simulink model "ad_pmsm_or"  (R2022b)
settings: Solver=FixedStepAuto  StartTime=0.0  StopTime=0.6  FixedStep=5e-7  MaxStep=1e-5  RelTol=1e-4
InitFcn:
  | Ts = 10e-6;
  | 
  | R = 0.958;
  | Ld = 5.25e-3;
  | Lq = 12e-3;
  | Pn = 4;
  | flux = 0.1827;
undefined symbols (not defined in the file): b0_d, DiscIntNeverNeededParam
libraries: simulink x12, slpidlib x7, spsPermanentMagnetSynchronousMachineLib x4, spsUniversalBridgeLib x4, spsDCVoltageSourceLib x4, powerlib_extras x2, sps_lib x1
(part 1 of 3)
settings Model: Creator=SUN  LastModifiedBy=崔波
settings SolverCC: ZeroCrossControl=DisableAll  AlgebraicLoopSolver=TrustRegion  AutoInsertRateTranBlk=on
settings DataIOCC: LimitDataPoints=on  SaveFormat=Array  SignalLoggingSaveFormat=ModelDataLogs  ReturnWorkspaceOutputs=off
settings OptimizationCC: ExpressionDepthLimit=2147483647  InitFltsAndDblsToZero=on  LifeSpan=inf
settings DebuggingCC: UnderspecifiedInitializationDetection=Classic  MergeDetectMultiDrivingBlocksExec=none  SolverPrmCheckMsg=warning  MultiTaskRateTransMsg=warning  FcnCallInpInsideContextMsg=warning  UnconnectedInputMsg=warning  UnconnectedOutputMsg=warning  UnconnectedLineMsg=warning  StateNameClashWarn=warning  SFUnexpectedBacktrackingDiag=warning  SFNoUnconditionalDefaultTransitionDiag=warning  SFExecutionAtInitializationDiag=none  SFMachineParentedDataDiag=warning  ArithmeticOperatorsInVariantConditions=warning
settings HardwareCC: ProdBitPerPointer=32  ProdBitPerSizeT=32  ProdBitPerPtrDiffT=32  ProdLargestAtomicFloat=None  ProdIntDivRoundTo=Undefined  ProdEndianess=Unspecified  ProdWordSize=32  ProdHWDeviceType=32-bit Generic
settings ModelReferenceCC: PropagateSignalLabelsOutOfModel=off
settings SFSimCC: SimUseLocalCustomCode=off  CustomCodeUndefinedFunction=UseInterfaceOnly
settings RTWCC: RTWUseLocalCustomCode=off
settings CodeAppCC: StateflowObjectComments=on
settings GRTTargetCC: TargetLangStandard=C89/C90 (ANSI)  CombineOutputUpdateFcns=off  GRTInterface=on
settings ConfigComp: CovMetricSettings=dw  CovSaveCumulativeToWorkspaceVar=on  CovSaveSingleToWorkspaceVar=on  CovExternalEMLEnable=off  CovSFcnEnable=off
settings SimscapeCC: SimscapeNormalizeSystem=off

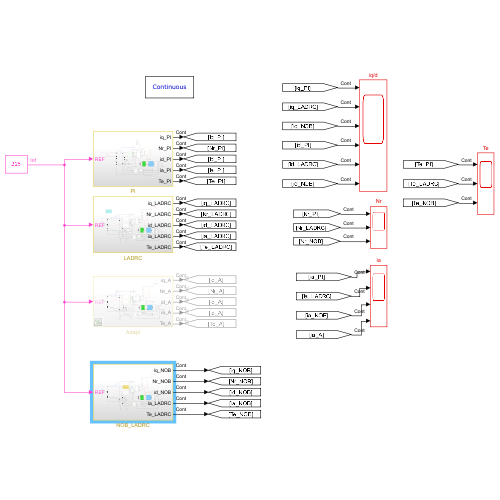
[thumbnail: Simulink's stored preview of the top-level diagram]
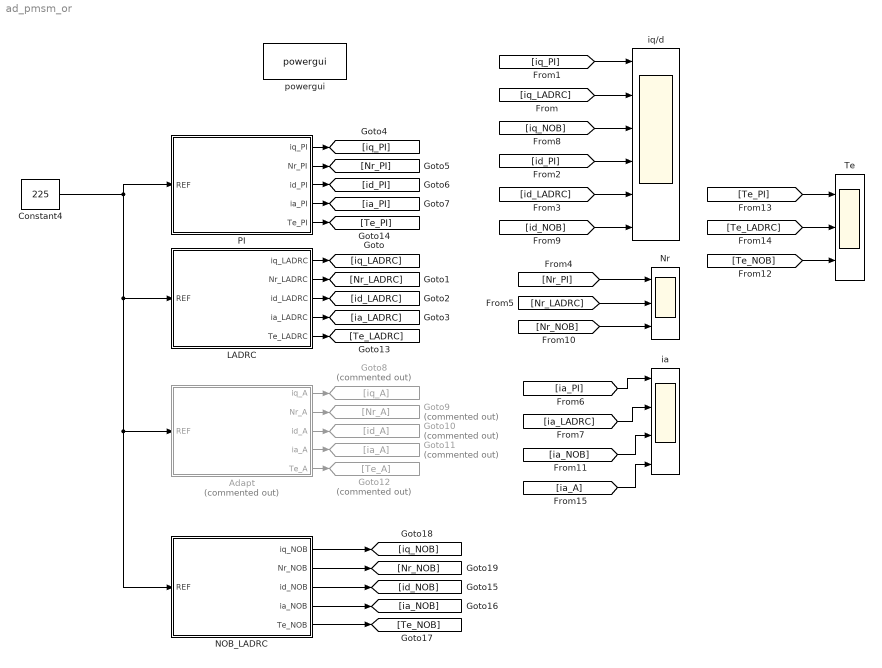
== system ad_pmsm_or ==
  Adapt : Subsystem  Commented=on
  Constant4 : Constant  Value=225
  Goto10 : Goto  Commented=on  GotoTag=id_A
  Goto11 : Goto  Commented=on  GotoTag=ia_A
  Goto12 : Goto  Commented=on  GotoTag=Te_A
  Goto8 : Goto  Commented=on  GotoTag=iq_A
  Goto9 : Goto  Commented=on  GotoTag=Nr_A
  LADRC : Subsystem
  NOB_LADRC : Subsystem
  Nr : Scope  NumInputPorts=3
  PI : Subsystem
  Te : Scope  NumInputPorts=3
  ia : Scope  NumInputPorts=4
  iq/d : Scope  NumInputPorts=6
  powergui : sps_lib/powergui  SimulationMode=Continuous  SampleTime=Ts  frequency=60  Iterations=50  frequencyindice=0  Pbase=100e6  ErrMax=1e-4  UnitsV=kV  UnitsW=MW  buscounter=0  FunctionMessages=off  echomessages=off  EnableUseOfTLC=off  CurrentSourceSwitches=on  DisableSnubberDevices=off  DisableRonSwitches=off  DisableVfSwitches=off  DisplayEquations=off  AutomaticDiscreteSolvers=off  SolverType=Tustin/Backward Euler (TBE)  Interpol=off  ExternalGateDelay=off  methode=off  Ts=0  x0status=blocks  SPID=off  SwTol=0  HookPort=off  NonlinearTolerance=1e-4  nMaxIteration=100  ContinueOnMaxIteration=off  RestoreLinks=warning  ResistiveCurrentMeasurement=off  Frange=[0:2:500]  Ylog=off  Xlog=on  ShowGrid=off  save=off  variable=ZData  structure=0  ZoomFFT=on  StartTime=0.0  cycles=1  DisplayStyle=1  fundamental=60  FreqAxis=off  MaxFrequency=1000  frequencyindicesteady=1  RmsSteady=1  display=off
  wires:
  LADRC/1(iq_LADRC) -> [iq_LADRC]
  LADRC/2(Nr_LADRC) -> [Nr_LADRC]
  LADRC/3(id_LADRC) -> [id_LADRC]
  LADRC/4(ia_LADRC) -> [ia_LADRC]
  [iq_PI] -> iq/d/1
  [id_PI] -> iq/d/4
  [id_LADRC] -> iq/d/5
  PI/2(Nr_PI) -> [Nr_PI]
  PI/4(ia_PI) -> [ia_PI]
  PI/3(id_PI) -> [id_PI]
  PI/1(iq_PI) -> [iq_PI]
  [Nr_PI] -> Nr/1
  [Nr_LADRC] -> Nr/2
  [ia_PI] -> ia/1
  [ia_LADRC] -> ia/2
  Adapt/2(Nr_A) -> Goto9/1
  Adapt/3(id_A) -> Goto10/1
  Constant4/1 -> NOB_LADRC/1(REF), Adapt/1(REF), LADRC/1(REF), PI/1(REF)
  Adapt/4(ia_A) -> Goto11/1
  Adapt/1(iq_A) -> Goto8/1
  [iq_NOB] -> iq/d/3
  [id_NOB] -> iq/d/6
  [Nr_NOB] -> Nr/3
  [ia_NOB] -> ia/3
  [Te_PI] -> Te/1
  [Te_LADRC] -> Te/2
  [Te_NOB] -> Te/3
  Adapt/5(Te_A) -> Goto12/1
  LADRC/5(Te_LADRC) -> [Te_LADRC]
  PI/5(Te_PI) -> [Te_PI]
  [iq_LADRC] -> iq/d/2
  NOB_LADRC/1(iq_NOB) -> [iq_NOB]
  NOB_LADRC/2(Nr_NOB) -> [Nr_NOB]
  NOB_LADRC/3(id_NOB) -> [id_NOB]
  NOB_LADRC/4(ia_NOB) -> [ia_NOB]
  NOB_LADRC/5(Te_NOB) -> [Te_NOB]
  [ia_A] -> ia/4

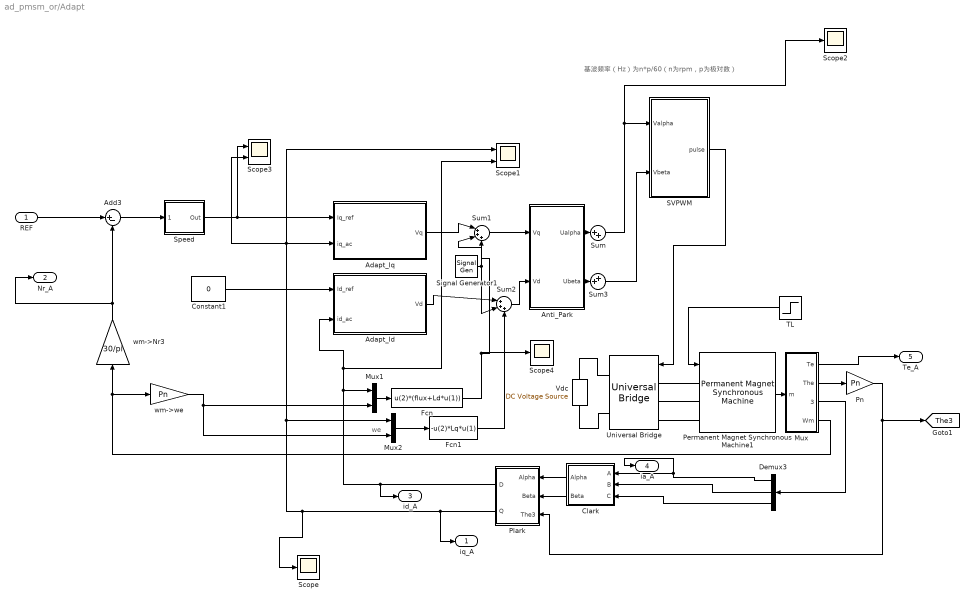
== system ad_pmsm_or/Adapt ==
  note: 基波频率（Hz）为n*p/60（n为rpm，p为极对数）
  note: we
  REF : Inport
  Adapt_Id : Subsystem  mask{Cd_l3=0.29, C_Krd=0.3, Ked=6.5, bd0=1/5.25e-3, wc_d=1100, wo_d=1100*3}
      mask DialogControl DescTextVar Prompt: 自适应谐振自抗扰控制器
      mask DialogControl ParameterGroupVar Prompt: 自抗扰控制器
      mask DialogControl Container3 Prompt: 自适应谐振控制器
      mask DialogControl Container4 Prompt: 频率自适应率
  Adapt_Iq : Subsystem  mask{bq0=1/12e-3, wc_q=1100, wo_q=1100*3, Cq_l3=0.29, C_Krq=0.3, Keq=0.3}
      mask DialogControl DescTextVar Prompt: 自适应谐振自抗扰控制器
      mask DialogControl ParameterGroupVar Prompt: 自抗扰控制器
      mask DialogControl Container3 Prompt: 自适应谐振控制器
      mask DialogControl Container4 Prompt: 频率自适应率
  Add3 : Sum  Inputs=|+-
  Anti_Park : Subsystem
  Clark : Subsystem
  Constant1 : Constant  Value=0
  Demux3 : Demux  Outputs=3
  Fcn : Fcn  Expr=u(2)*(flux+Ld*u(1))
  Fcn1 : Fcn  Expr=-u(2)*Lq*u(1)
  Mux : Subsystem
  Mux1 : Mux  Inputs=2
  Mux2 : Mux  Inputs=2
  Permanent Magnet Synchronous Machine1 : spsPermanentMagnetSynchronousMachineLib/Permanent Magnet Synchronous Machine  NbPhases=3  FluxDistribution=Sinusoidal  RotorType=Salient-pole  MechanicalLoad=Torque Tm  PresetModel=No  ShowDetailedParameters=on  MeasurementBus=off  Resistance=0.958  Inductance=8.5e-3  dqInductances=[5.25e-3,12e-3]  La=0.000835  MachineConstant=Flux linkage established by magnets (V.s)  Flux=0.1827  VoltageCst=132.5525  TorqueCst=1.0962  Flat=120  Mechanical=[0.003 0.008 4]  PolePairs=3  InitialConditions=[0,0, 0,0]  InitialConditions5ph=[0 0 0 0 0 0]  RefAngle=Aligned with phase A axis (original Park)  IterativeDiscreteModel=Trapezoidal non iterative  TsBlock=-1  TsPowergui=0
  Plark : Subsystem
  Pn : Gain  Gain=Pn
  SVPWM : Subsystem
  Scope : Scope
  Scope1 : Scope  NumInputPorts=2
  Scope2 : Scope
  Scope3 : Scope  NumInputPorts=2
  Scope4 : Scope
  Signal Generator1 : SignalGenerator  Amplitude=5*0.5  Frequency=90
  Speed : Subsystem  AncestorBlock=|  DialogController=POWERSYS.PowerSysDialog  mask(Discrete PI Controller){Kpw=0.06, Kiw=3, Ba=0, Par_Limits=[30 -30], Init=0, Ts=1e-3}
      | powerlib_extras/Discrete 
      | Control Blocks/Discrete
      | PI Controller
      mask prompts: Kpw "Proportional gain (Kp):"; Kiw "Integral gain (Ki):"; Ba "feedback gain (Ba)"; Par_Limits "Output limits: [ Upper   Lower ]"; Init "Output initial value:"; Ts "Sample time:"
      mask help: This block implements a discrete PI controller.
      mask init:
      | UpperLimit=Par_Limits(1);
      | LowerLimit=Par_Limits(2);
      | power_initmask();
      settings: LibrarySourceBlock=|
      | powerlib_extras/Discrete
      | Control Blocks/Discrete
      | PI Controller
      mask Help: This block is part of a subset of blocks in the Extras library that does not have documentation associated with it, other than the block mask description.
      mask Display: disp('PI');
  Sum : Sum  Inputs=|++
  Sum1 : Sum  Inputs=|+++
  Sum2 : Sum  Inputs=|+++
  Sum3 : Sum  Inputs=++|
  TL : Step  Time=0  After=5  SampleTime=0
  Universal Bridge : spsUniversalBridgeLib/Universal Bridge  Arms=3  SnubberResistance=1e5  SnubberCapacitance=inf  Device=IGBT / Diodes  Ron=1e-3  Lon=0  ForwardVoltages="[  0  0  ]"  ForwardVoltage=0  GTOparameters=[ 10e-6 , 20e-6 ]  IGBTparameters=[ 1e-6 , 2e-6 ]  Measurements=None  Measurements_2=None  converterType=Rectifier
  Vdc : spsDCVoltageSourceLib/DC Voltage Source  Amplitude=311  Measurements=None
  wm->Nr3 : Gain  Gain=30/pi
  wm->we : Gain  Gain=Pn
  iq_A : Outport
  Nr_A : Outport  Port=2
  id_A : Outport  Port=3
  ia_A : Outport  Port=4
  Te_A : Outport  Port=5
  tag scope: The3=global
  wires:
  Clark/1(Alpha) -> Plark/1(Alpha)
  TL/1 -> Permanent Magnet Synchronous Machine1/1
  Permanent Magnet Synchronous Machine1/1 -> Mux/1(m)
  wm->Nr3/1 -> Nr_A/1, Add3/2
  Mux/4(Wm) -> wm->we/1, wm->Nr3/1
  Add3/1 -> Speed/1(Error)
  SVPWM/1(pulse) -> Universal Bridge/1
  Mux/3(Iabc2) -> Demux3/1
  Clark/2(Beta) -> Plark/2(Beta)
  REF/1 -> Add3/1
  Mux/2(The) -> Pn/1
  Plark/1(D) -> id_A/1, Mux1/1, Adapt_Id/2(id_ac), Scope1/2
  Pn/1 -> [The3], Plark/3(The3)
  Speed/1(Out) -> Scope3/1, Adapt_Iq/1(Iq_ref)
  Plark/2(Q) -> Scope/1, Scope3/2, Scope1/1, Adapt_Iq/2(iq_ac), Mux2/1, iq_A/1
  wm->we/1 -> Mux2/2, Mux1/2
  Mux2/1 -> Fcn1/1
  Mux1/1 -> Fcn/1
  Adapt_Iq/1(Vq) -> Sum1/1
  Sum1/1 -> Anti_Park/1(Vq)
  Fcn/1 -> Sum1/3, Scope4/1
  Adapt_Id/1(Vd) -> Sum2/1
  Sum2/1 -> Anti_Park/2(Vd)
  Sum/1 -> Scope2/1, SVPWM/1(Valpha)
  Anti_Park/2(Ubeta) -> Sum3/2
  Sum3/1 -> SVPWM/2(Vbeta)
  Anti_Park/1(Ualpha) -> Sum/1
  Constant1/1 -> Adapt_Id/1(Id_ref)
  Mux/1(Te) -> Te_A/1
  Demux3/1 -> ia_A/1, Clark/1(A)
  Demux3/2 -> Clark/2(B)
  Demux3/3 -> Clark/3(C)
  Signal Generator1/1 -> Sum1/2, Sum2/2
  Fcn1/1 -> Sum2/3
  connections:
  Permanent Magnet Synchronous Machine1/LConn3 -- Universal Bridge/LConn3
  Universal Bridge/RConn2 -- Vdc/LConn1
  Permanent Magnet Synchronous Machine1/LConn2 -- Universal Bridge/LConn2
  Universal Bridge/RConn1 -- Vdc/RConn1
  Universal Bridge/LConn1 -- Permanent Magnet Synchronous Machine1/LConn1

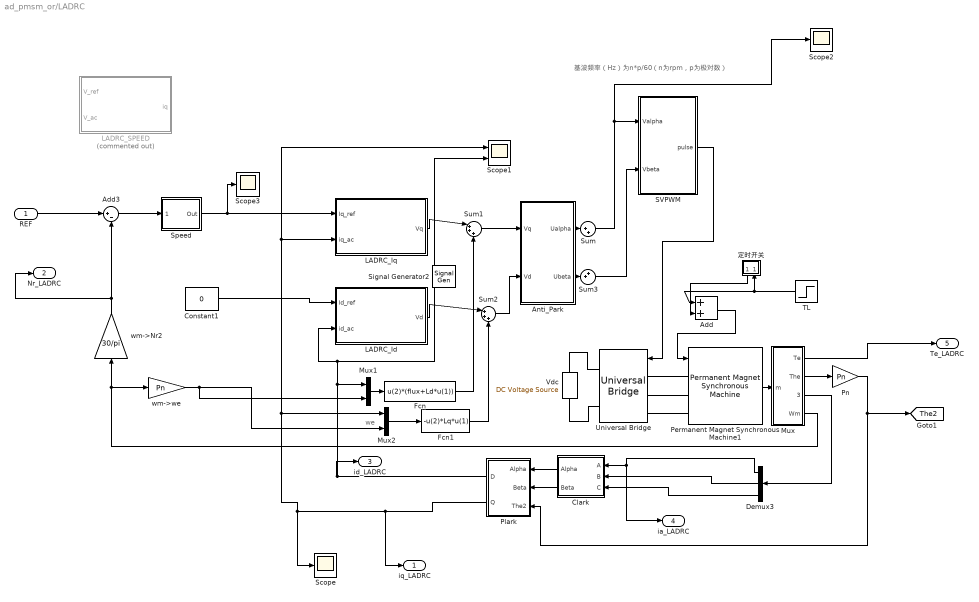
== system ad_pmsm_or/LADRC ==
  note: 基波频率（Hz）为n*p/60（n为rpm，p为极对数）
  note: we
  REF : Inport
  Add : Sum
  Add3 : Sum  Inputs=|+-
  Anti_Park : Subsystem
  Clark : Subsystem
  Constant1 : Constant  Value=0
  Demux3 : Demux  Outputs=3
  Fcn : Fcn  Expr=u(2)*(flux+Ld*u(1))
  Fcn1 : Fcn  Expr=-u(2)*Lq*u(1)
  LADRC_Id : Subsystem  mask{b0_d=1/5.25e-3, wc_d=1100, wo_d=1.5*1100}
      mask DialogControl ParameterGroupVar Prompt: 参数
  LADRC_Iq : Subsystem  mask{b0_q=1/12e-3, wc_q=1100, wo_q=1.5*1100}
      mask DialogControl ParameterGroupVar Prompt: 参数
  LADRC_SPEED : Subsystem  Commented=on  mask{b0_V=1/5.25e-3, wc_V=30, wo_V=150}
      mask DialogControl ParameterGroupVar Prompt: 参数
  Mux : Subsystem
  Mux1 : Mux  Inputs=2
  Mux2 : Mux  Inputs=2
  Permanent Magnet Synchronous Machine1 : spsPermanentMagnetSynchronousMachineLib/Permanent Magnet Synchronous Machine  NbPhases=3  FluxDistribution=Sinusoidal  RotorType=Salient-pole  MechanicalLoad=Torque Tm  PresetModel=No  ShowDetailedParameters=on  MeasurementBus=off  Resistance=0.958  Inductance=8.5e-3  dqInductances=[5.25e-3,12e-3]  La=0.000835  MachineConstant=Flux linkage established by magnets (V.s)  Flux=0.1827  VoltageCst=132.5525  TorqueCst=1.0962  Flat=120  Mechanical=[0.003 0.008 4]  PolePairs=3  InitialConditions=[0,0, 0,0]  InitialConditions5ph=[0 0 0 0 0 0]  RefAngle=Aligned with phase A axis (original Park)  IterativeDiscreteModel=Trapezoidal non iterative  TsBlock=-1  TsPowergui=0
  Plark : Subsystem
  Pn : Gain  Gain=Pn
  SVPWM : Subsystem
  Scope : Scope
  Scope1 : Scope  NumInputPorts=2
  Scope2 : Scope
  Scope3 : Scope
  Signal Generator2 : SignalGenerator  Amplitude=5*0.5  Frequency=90
  Speed : Subsystem  AncestorBlock=|  DialogController=POWERSYS.PowerSysDialog  mask(Discrete PI Controller){Kpw=0.06, Kiw=3, Ba=0, Par_Limits=[30 -30], Init=0, Ts=1e-3}
      | powerlib_extras/Discrete 
      | Control Blocks/Discrete
      | PI Controller
      mask prompts: Kpw "Proportional gain (Kp):"; Kiw "Integral gain (Ki):"; Ba "feedback gain (Ba)"; Par_Limits "Output limits: [ Upper   Lower ]"; Init "Output initial value:"; Ts "Sample time:"
      mask help: This block implements a discrete PI controller.
      mask init:
      | UpperLimit=Par_Limits(1);
      | LowerLimit=Par_Limits(2);
      | power_initmask();
      settings: LibrarySourceBlock=|
      | powerlib_extras/Discrete
      | Control Blocks/Discrete
      | PI Controller
      mask Help: This block is part of a subset of blocks in the Extras library that does not have documentation associated with it, other than the block mask description.
      mask Display: disp('PI');
  Sum : Sum  Inputs=|++
  Sum1 : Sum  Inputs=|+++
  Sum2 : Sum  Inputs=|+++
  Sum3 : Sum  Inputs=++|
  TL : Step  Time=0  After=5  SampleTime=0
  Universal Bridge : spsUniversalBridgeLib/Universal Bridge  Arms=3  SnubberResistance=1e5  SnubberCapacitance=inf  Device=IGBT / Diodes  Ron=1e-3  Lon=0  ForwardVoltages="[  0  0  ]"  ForwardVoltage=0  GTOparameters=[ 10e-6 , 20e-6 ]  IGBTparameters=[ 1e-6 , 2e-6 ]  Measurements=None  Measurements_2=None  converterType=Rectifier
  Vdc : spsDCVoltageSourceLib/DC Voltage Source  Amplitude=311  Measurements=None
  wm->Nr2 : Gain  Gain=30/pi
  wm->we : Gain  Gain=Pn
  定时开关 : Subsystem
      settings: PortSchema="{\"entries\":[{\"content\":{\"sides\":[{\"content\":{\"connectorIds\":[]},\"type\":\"ConnectorPlacement.EquallySpacedRectSide\",\"uuid\":\"3d2fe186-dc42-49ec-885f-99f75e378e5c\"},{\"content\":{\"connectorIds\":[\"Out1\",\"In1\"],\"side\":\"RIGHT\"},\"type\":\"ConnectorPlacement.EquallySpacedRectSide\",\"uuid\":\"6078a930-c81b-430f-bb15-8ce430174df2\"},{\"content\":{\"connectorIds\":[],\"side\":\"TOP\"},\"type\":\"ConnectorPlacement.EquallySpacedRectSide\",\"uuid\":\"3cfcb01b-8519-4e61-acfc-4433e819e8a6\"},{\"content\":{\"connectorIds\":[],\"side\":\"BOTTOM\"},\"type\":\"ConnectorPlacement.EquallySpacedRectSide\",\"uuid\":\"a8c23dbb-c537-4582-83a4-36b1febadf31\"}]},\"type\":\"ConnectorPlacement.EquallySpacedConnector\",\"uuid\":\"a7464e76-cd29-42ec-8ed6-de6b90538fe1\"}],\"packageUris\":[\"http://schema.mathworks.com/mf0/Connector/R2020b\"],\"version\":\"1.0\"}"
  iq_LADRC : Outport
  Nr_LADRC : Outport  Port=2
  id_LADRC : Outport  Port=3
  ia_LADRC : Outport  Port=4
  Te_LADRC : Outport  Port=5
  tag scope: The2=global
  wires:
  Clark/1(Alpha) -> Plark/1(Alpha)
  Permanent Magnet Synchronous Machine1/1 -> Mux/1(m)
  wm->Nr2/1 -> Nr_LADRC/1, Add3/2
  Mux/4(Wm) -> wm->we/1, wm->Nr2/1
  Add3/1 -> Speed/1(Error)
  SVPWM/1(pulse) -> Universal Bridge/1
  Mux/3(Iabc2) -> Demux3/1
  Clark/2(Beta) -> Plark/2(Beta)
  REF/1 -> Add3/1
  Mux/2(The) -> Pn/1
  Constant1/1 -> LADRC_Id/1(Id_ref)
  Plark/1(D) -> id_LADRC/1, Mux1/1, Scope1/2, LADRC_Id/2(id_ac)
  Pn/1 -> [The2], Plark/3(The2)
  Speed/1(Out) -> Scope3/1, LADRC_Iq/1(Iq_ref)
  Plark/2(Q) -> Scope1/1, LADRC_Iq/2(iq_ac), Mux2/1, Scope/1, iq_LADRC/1
  wm->we/1 -> Mux2/2, Mux1/2
  Mux2/1 -> Fcn1/1
  Mux1/1 -> Fcn/1
  LADRC_Iq/1(Vq) -> Sum1/1
  Sum1/1 -> Anti_Park/1(Vq)
  LADRC_Id/1(Vd) -> Sum2/1
  Sum2/1 -> Anti_Park/2(Vd)
  Sum/1 -> Scope2/1, SVPWM/1(Valpha)
  Anti_Park/2(Ubeta) -> Sum3/2
  Sum3/1 -> SVPWM/2(Vbeta)
  Anti_Park/1(Ualpha) -> Sum/1
  Mux/1(Te) -> Te_LADRC/1
  Demux3/3 -> Clark/3(C)
  Demux3/1 -> ia_LADRC/1, Clark/1(A)
  Demux3/2 -> Clark/2(B)
  Fcn1/1 -> Sum2/3
  Fcn/1 -> Sum1/3
  ? -> ?
  定时开关/1(Out1) -> Add/2
  TL/1 -> Add/1, 定时开关/1(In1)
  Add/1 -> Permanent Magnet Synchronous Machine1/1
  connections:
  Permanent Magnet Synchronous Machine1/LConn3 -- Universal Bridge/LConn3
  Universal Bridge/RConn2 -- Vdc/LConn1
  Permanent Magnet Synchronous Machine1/LConn2 -- Universal Bridge/LConn2
  Universal Bridge/RConn1 -- Vdc/RConn1
  Universal Bridge/LConn1 -- Permanent Magnet Synchronous Machine1/LConn1

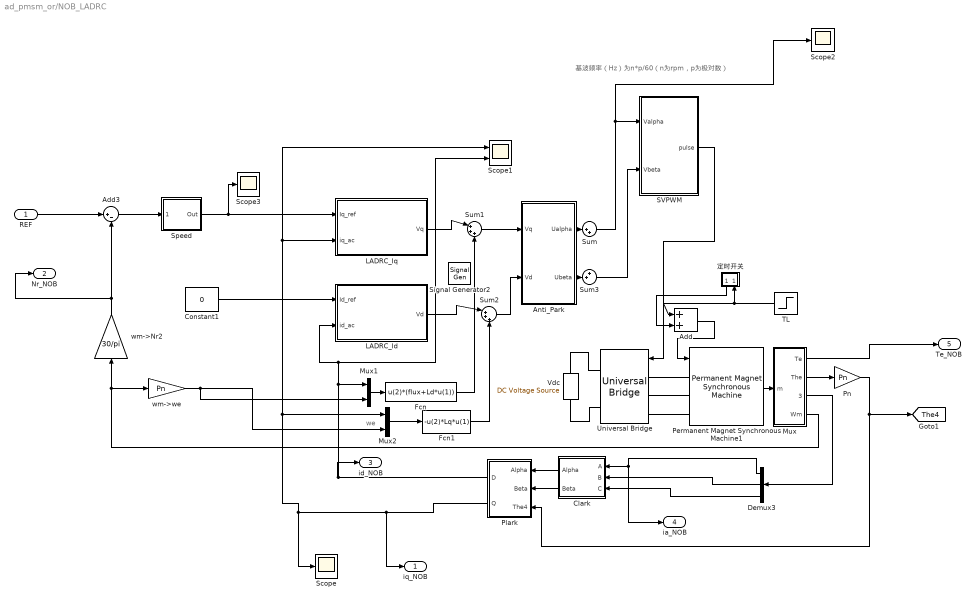
== system ad_pmsm_or/NOB_LADRC ==
  note: 基波频率（Hz）为n*p/60（n为rpm，p为极对数）
  note: we
  REF : Inport
  Add : Sum
  Add3 : Sum  Inputs=|+-
  Anti_Park : Subsystem
  Clark : Subsystem
  Constant1 : Constant  Value=0
  Demux3 : Demux  Outputs=3
  Fcn : Fcn  Expr=u(2)*(flux+Ld*u(1))
  Fcn1 : Fcn  Expr=-u(2)*Lq*u(1)
  LADRC_Id : Subsystem  mask{b0_d=1/5.25e-3, wc_d=1100, wo_d=1.5*1100}
      mask DialogControl ParameterGroupVar Prompt: 参数
  LADRC_Iq : Subsystem  mask{b0_q=1/12e-3, wc_q=1100, wo_q=1.5*1100}
      mask DialogControl ParameterGroupVar Prompt: 参数
  Mux : Subsystem
  Mux1 : Mux  Inputs=2
  Mux2 : Mux  Inputs=2
  Permanent Magnet Synchronous Machine1 : spsPermanentMagnetSynchronousMachineLib/Permanent Magnet Synchronous Machine  NbPhases=3  FluxDistribution=Sinusoidal  RotorType=Salient-pole  MechanicalLoad=Torque Tm  PresetModel=No  ShowDetailedParameters=on  MeasurementBus=off  Resistance=0.958  Inductance=8.5e-3  dqInductances=[5.25e-3,12e-3]  La=0.000835  MachineConstant=Flux linkage established by magnets (V.s)  Flux=0.1827  VoltageCst=132.5525  TorqueCst=1.0962  Flat=120  Mechanical=[0.003 0.008 4]  PolePairs=3  InitialConditions=[0,0, 0,0]  InitialConditions5ph=[0 0 0 0 0 0]  RefAngle=Aligned with phase A axis (original Park)  IterativeDiscreteModel=Trapezoidal non iterative  TsBlock=-1  TsPowergui=0
  Plark : Subsystem
  Pn : Gain  Gain=Pn
  SVPWM : Subsystem
  Scope : Scope
  Scope1 : Scope  NumInputPorts=2
  Scope2 : Scope
  Scope3 : Scope
  Signal Generator2 : SignalGenerator  Amplitude=5*0.5  Frequency=90
  Speed : Subsystem  AncestorBlock=|  DialogController=POWERSYS.PowerSysDialog  mask(Discrete PI Controller){Kpw=0.06, Kiw=3, Ba=0, Par_Limits=[30 -30], Init=0, Ts=1e-3}
      | powerlib_extras/Discrete 
      | Control Blocks/Discrete
      | PI Controller
      mask prompts: Kpw "Proportional gain (Kp):"; Kiw "Integral gain (Ki):"; Ba "feedback gain (Ba)"; Par_Limits "Output limits: [ Upper   Lower ]"; Init "Output initial value:"; Ts "Sample time:"
      mask help: This block implements a discrete PI controller.
      mask init:
      | UpperLimit=Par_Limits(1);
      | LowerLimit=Par_Limits(2);
      | power_initmask();
      settings: LibrarySourceBlock=|
      | powerlib_extras/Discrete
      | Control Blocks/Discrete
      | PI Controller
      mask Help: This block is part of a subset of blocks in the Extras library that does not have documentation associated with it, other than the block mask description.
      mask Display: disp('PI');
  Sum : Sum  Inputs=|++
  Sum1 : Sum  Inputs=|+++
  Sum2 : Sum  Inputs=|+++
  Sum3 : Sum  Inputs=++|
  TL : Step  Time=0  After=5  SampleTime=0
  Universal Bridge : spsUniversalBridgeLib/Universal Bridge  Arms=3  SnubberResistance=1e5  SnubberCapacitance=inf  Device=IGBT / Diodes  Ron=1e-3  Lon=0  ForwardVoltages="[  0  0  ]"  ForwardVoltage=0  GTOparameters=[ 10e-6 , 20e-6 ]  IGBTparameters=[ 1e-6 , 2e-6 ]  Measurements=None  Measurements_2=None  converterType=Rectifier
  Vdc : spsDCVoltageSourceLib/DC Voltage Source  Amplitude=311  Measurements=None
  wm->Nr2 : Gain  Gain=30/pi
  wm->we : Gain  Gain=Pn
  定时开关 : Subsystem
      settings: PortSchema="{\"entries\":[{\"content\":{\"sides\":[{\"content\":{\"connectorIds\":[]},\"type\":\"ConnectorPlacement.EquallySpacedRectSide\",\"uuid\":\"3d2fe186-dc42-49ec-885f-99f75e378e5c\"},{\"content\":{\"connectorIds\":[\"Out1\",\"In1\"],\"side\":\"RIGHT\"},\"type\":\"ConnectorPlacement.EquallySpacedRectSide\",\"uuid\":\"6078a930-c81b-430f-bb15-8ce430174df2\"},{\"content\":{\"connectorIds\":[],\"side\":\"TOP\"},\"type\":\"ConnectorPlacement.EquallySpacedRectSide\",\"uuid\":\"3cfcb01b-8519-4e61-acfc-4433e819e8a6\"},{\"content\":{\"connectorIds\":[],\"side\":\"BOTTOM\"},\"type\":\"ConnectorPlacement.EquallySpacedRectSide\",\"uuid\":\"a8c23dbb-c537-4582-83a4-36b1febadf31\"}]},\"type\":\"ConnectorPlacement.EquallySpacedConnector\",\"uuid\":\"a7464e76-cd29-42ec-8ed6-de6b90538fe1\"}],\"packageUris\":[\"http://schema.mathworks.com/mf0/Connector/R2020b\"],\"version\":\"1.0\"}"
  iq_NOB : Outport
  Nr_NOB : Outport  Port=2
  id_NOB : Outport  Port=3
  ia_NOB : Outport  Port=4
  Te_NOB : Outport  Port=5
  tag scope: The4=global
  wires:
  Clark/1(Alpha) -> Plark/1(Alpha)
  Permanent Magnet Synchronous Machine1/1 -> Mux/1(m)
  wm->Nr2/1 -> Nr_NOB/1, Add3/2
  Mux/4(Wm) -> wm->we/1, wm->Nr2/1
  Add3/1 -> Speed/1(Error)
  SVPWM/1(pulse) -> Universal Bridge/1
  Mux/3(Iabc2) -> Demux3/1
  Clark/2(Beta) -> Plark/2(Beta)
  REF/1 -> Add3/1
  Mux/2(The) -> Pn/1
  Constant1/1 -> LADRC_Id/1(Id_ref)
  Plark/1(D) -> id_NOB/1, Mux1/1, Scope1/2, LADRC_Id/2(id_ac)
  Pn/1 -> [The4], Plark/3(The4)
  Speed/1(Out) -> Scope3/1, LADRC_Iq/1(Iq_ref)
  Plark/2(Q) -> Scope1/1, LADRC_Iq/2(iq_ac), Mux2/1, Scope/1, iq_NOB/1
  wm->we/1 -> Mux2/2, Mux1/2
  Mux2/1 -> Fcn1/1
  Mux1/1 -> Fcn/1
  LADRC_Iq/1(Vq) -> Sum1/1
  Sum1/1 -> Anti_Park/1(Vq)
  LADRC_Id/1(Vd) -> Sum2/1
  Sum2/1 -> Anti_Park/2(Vd)
  Sum/1 -> Scope2/1, SVPWM/1(Valpha)
  Anti_Park/2(Ubeta) -> Sum3/2
  Sum3/1 -> SVPWM/2(Vbeta)
  Anti_Park/1(Ualpha) -> Sum/1
  Mux/1(Te) -> Te_NOB/1
  Demux3/3 -> Clark/3(C)
  Demux3/1 -> ia_NOB/1, Clark/1(A)
  Demux3/2 -> Clark/2(B)
  Fcn/1 -> Sum1/3
  Fcn1/1 -> Sum2/3
  Add/1 -> Permanent Magnet Synchronous Machine1/1
  TL/1 -> 定时开关/1(In1), Add/1
  定时开关/1(Out1) -> Add/2
  connections:
  Permanent Magnet Synchronous Machine1/LConn3 -- Universal Bridge/LConn3
  Universal Bridge/RConn2 -- Vdc/LConn1
  Permanent Magnet Synchronous Machine1/LConn2 -- Universal Bridge/LConn2
  Universal Bridge/RConn1 -- Vdc/RConn1
  Universal Bridge/LConn1 -- Permanent Magnet Synchronous Machine1/LConn1

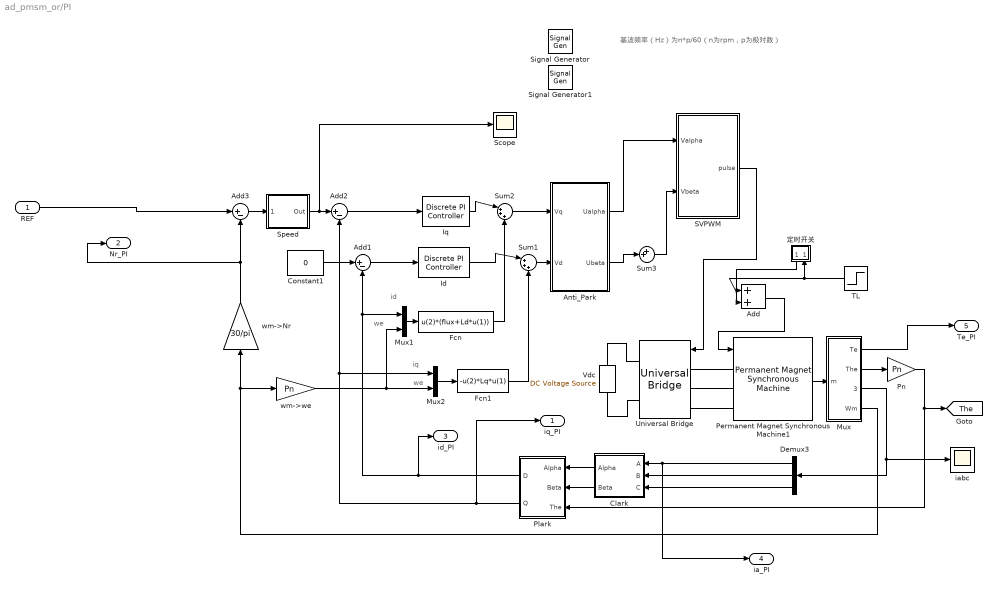
== system ad_pmsm_or/PI ==
  note: iq
  note: we
  note: we
  note: id
  note: 基波频率（Hz）为n*p/60（n为rpm，p为极对数）
  REF : Inport
  Add : Sum
  Add1 : Sum  Inputs=|+-
  Add2 : Sum  Inputs=|+-
  Add3 : Sum  Inputs=|+-
  Anti_Park : Subsystem
  Clark : Subsystem
  Constant1 : Constant  Value=0
  Demux3 : Demux  Outputs=3
  Fcn : Fcn  Expr=u(2)*(flux+Ld*u(1))
  Fcn1 : Fcn  Expr=-u(2)*Lq*u(1)
  Id : powerlib_extras/Discrete  Control Blocks/Discrete PI Controller  Kp=Ld*1100  Ki=R*1100  Par_Limits=[311*0.9*sqrt(1/3) -311*0.9*sqrt(1/3)]  Init=0  Ts=1e-4
  Iq : powerlib_extras/Discrete  Control Blocks/Discrete PI Controller  Kp=Lq*1100  Ki=R*1100  Par_Limits=[311*0.9*sqrt(1/3) -311*0.9*sqrt(1/3)]  Init=0  Ts=1e-4
  Mux : Subsystem
  Mux1 : Mux  Inputs=2
  Mux2 : Mux  Inputs=2
  Permanent Magnet Synchronous Machine1 : spsPermanentMagnetSynchronousMachineLib/Permanent Magnet Synchronous Machine  NbPhases=3  FluxDistribution=Sinusoidal  RotorType=Salient-pole  MechanicalLoad=Torque Tm  PresetModel=No  ShowDetailedParameters=on  MeasurementBus=off  Resistance=0.958  Inductance=8.5e-3  dqInductances=[5.25e-3,12e-3]  La=0.000835  MachineConstant=Flux linkage established by magnets (V.s)  Flux=0.1827  VoltageCst=132.5525  TorqueCst=1.0962  Flat=120  Mechanical=[0.003 0.008 4]  PolePairs=3  InitialConditions=[0,0, 0,0]  InitialConditions5ph=[0 0 0 0 0 0]  RefAngle=Aligned with phase A axis (original Park)  IterativeDiscreteModel=Trapezoidal non iterative  TsBlock=-1  TsPowergui=0
  Plark : Subsystem
  Pn : Gain  Gain=Pn
  SVPWM : Subsystem
  Scope : Scope
  Signal Generator : SignalGenerator  Amplitude=109*0.05  Frequency=1000*4/60*5
  Signal Generator1 : SignalGenerator  Amplitude=5*0.5  Frequency=90
  Speed : Subsystem  AncestorBlock=|  DialogController=POWERSYS.PowerSysDialog  mask(Discrete PI Controller){Kpw=0.06, Kiw=3, Ba=0, Par_Limits=[30 -30], Init=0, Ts=1e-3}
      | powerlib_extras/Discrete 
      | Control Blocks/Discrete
      | PI Controller
      mask prompts: Kpw "Proportional gain (Kp):"; Kiw "Integral gain (Ki):"; Ba "feedback gain (Ba)"; Par_Limits "Output limits: [ Upper   Lower ]"; Init "Output initial value:"; Ts "Sample time:"
      mask help: This block implements a discrete PI controller.
      mask init:
      | UpperLimit=Par_Limits(1);
      | LowerLimit=Par_Limits(2);
      | power_initmask();
      settings: LibrarySourceBlock=|
      | powerlib_extras/Discrete
      | Control Blocks/Discrete
      | PI Controller
      mask Help: This block is part of a subset of blocks in the Extras library that does not have documentation associated with it, other than the block mask description.
      mask Display: disp('PI');
  Sum1 : Sum  Inputs=|+++
  Sum2 : Sum  Inputs=|+++
  Sum3 : Sum  Inputs=++|
  TL : Step  Time=0  After=5  SampleTime=0
  Universal Bridge : spsUniversalBridgeLib/Universal Bridge  Arms=3  SnubberResistance=1e5  SnubberCapacitance=inf  Device=IGBT / Diodes  Ron=1e-3  Lon=0  ForwardVoltages="[  0  0  ]"  ForwardVoltage=0  GTOparameters=[ 10e-6 , 20e-6 ]  IGBTparameters=[ 1e-6 , 2e-6 ]  Measurements=None  Measurements_2=None  converterType=Rectifier
  Vdc : spsDCVoltageSourceLib/DC Voltage Source  Amplitude=311  Measurements=None
  iabc : Scope
  wm->Nr : Gain  Gain=30/pi
  wm->we : Gain  Gain=Pn
  定时开关 : Subsystem
      settings: PortSchema="{\"entries\":[{\"content\":{\"sides\":[{\"content\":{\"connectorIds\":[]},\"type\":\"ConnectorPlacement.EquallySpacedRectSide\",\"uuid\":\"3d2fe186-dc42-49ec-885f-99f75e378e5c\"},{\"content\":{\"connectorIds\":[\"Out1\",\"In1\"],\"side\":\"RIGHT\"},\"type\":\"ConnectorPlacement.EquallySpacedRectSide\",\"uuid\":\"6078a930-c81b-430f-bb15-8ce430174df2\"},{\"content\":{\"connectorIds\":[],\"side\":\"TOP\"},\"type\":\"ConnectorPlacement.EquallySpacedRectSide\",\"uuid\":\"3cfcb01b-8519-4e61-acfc-4433e819e8a6\"},{\"content\":{\"connectorIds\":[],\"side\":\"BOTTOM\"},\"type\":\"ConnectorPlacement.EquallySpacedRectSide\",\"uuid\":\"a8c23dbb-c537-4582-83a4-36b1febadf31\"}]},\"type\":\"ConnectorPlacement.EquallySpacedConnector\",\"uuid\":\"a7464e76-cd29-42ec-8ed6-de6b90538fe1\"}],\"packageUris\":[\"http://schema.mathworks.com/mf0/Connector/R2020b\"],\"version\":\"1.0\"}"
  iq_PI : Outport
  Nr_PI : Outport  Port=2
  id_PI : Outport  Port=3
  ia_PI : Outport  Port=4
  Te_PI : Outport  Port=5
  tag scope: The=global
  wires:
  Clark/1(Alpha) -> Plark/1(Alpha)
  Mux1/1 -> Fcn/1
  Add1/1 -> Id/1
  Permanent Magnet Synchronous Machine1/1 -> Mux/1(m)
  wm->Nr/1 -> Nr_PI/1, Add3/2
  Mux/4(Wm) -> wm->we/1, wm->Nr/1
  Mux2/1 -> Fcn1/1
  Sum2/1 -> Anti_Park/1(Vq)
  Add3/1 -> Speed/1(Error)
  Plark/2(Q) -> iq_PI/1, Mux2/1, Add2/2
  wm->we/1 -> Mux2/2, Mux1/2
  Pn/1 -> Plark/3(The), [The]
  Add2/1 -> Iq/1
  Id/1 -> Sum1/1
  Sum1/1 -> Anti_Park/2(Vd)
  SVPWM/1(pulse) -> Universal Bridge/1
  Iq/1 -> Sum2/1
  Plark/1(D) -> id_PI/1, Mux1/1, Add1/2
  Mux/3(Iabc) -> iabc/1, Demux3/1
  Clark/2(Beta) -> Plark/2(Beta)
  REF/1 -> Add3/1
  Mux/2(The) -> Pn/1
  Constant1/1 -> Add1/1
  Speed/1(Out) -> Scope/1, Add2/1
  Anti_Park/1(Ualpha) -> SVPWM/1(Valpha)
  Anti_Park/2(Ubeta) -> Sum3/2
  Sum3/1 -> SVPWM/2(Vbeta)
  Mux/1(Te) -> Te_PI/1
  Demux3/1 -> ia_PI/1, Clark/1(A)
  Demux3/2 -> Clark/2(B)
  Demux3/3 -> Clark/3(C)
  Fcn/1 -> Sum2/3
  Fcn1/1 -> Sum1/3
  定时开关/1(Out1) -> Add/2
  TL/1 -> Add/1, 定时开关/1(In1)
  Add/1 -> Permanent Magnet Synchronous Machine1/1
  connections:
  Permanent Magnet Synchronous Machine1/LConn1 -- Universal Bridge/LConn1
  Permanent Magnet Synchronous Machine1/LConn3 -- Universal Bridge/LConn3
  Universal Bridge/RConn2 -- Vdc/LConn1
  Permanent Magnet Synchronous Machine1/LConn2 -- Universal Bridge/LConn2
  Universal Bridge/RConn1 -- Vdc/RConn1

== system ad_pmsm_or/Adapt/Adapt_Id ==
  Id_ref : Inport
  id_ac : Inport  Port=2
  A_LESO : Subsystem
  Gain1 : Gain  Gain=1/bd0
  NLESF : Subsystem
      settings: PortSchema="{\"entries\":[{\"content\":{\"sides\":[{\"content\":{\"connectorIds\":[]},\"type\":\"ConnectorPlacement.EquallySpacedRectSide\",\"uuid\":\"855ad99d-f275-44e1-8b5b-56b977b466e8\"},{\"content\":{\"connectorIds\":[],\"side\":\"RIGHT\"},\"type\":\"ConnectorPlacement.EquallySpacedRectSide\",\"uuid\":\"4b878b09-ea31-423b-8484-bd272f0e87c8\"},{\"content\":{\"connectorIds\":[\"In1\"],\"side\":\"TOP\"},\"type\":\"ConnectorPlacement.EquallySpacedRectSide\",\"uuid\":\"57c50dd4-c343-4c9b-a4ed-e8a0ac5e39c8\"},{\"content\":{\"connectorIds\":[\"Out1\"],\"side\":\"BOTTOM\"},\"type\":\"ConnectorPlacement.EquallySpacedRectSide\",\"uuid\":\"ac7a5b07-13b6-4023-b74a-bbacaa2441c8\"}]},\"type\":\"ConnectorPlacement.EquallySpacedConnector\",\"uuid\":\"c498a5af-adea-4d67-ae4d-0db2496b6d76\"}],\"packageUris\":[\"http://schema.mathworks.com/mf0/Connector/R2020b\"],\"version\":\"1.0\"}"
  NOB : Subsystem
      settings: PortSchema="{\"entries\":[{\"content\":{\"sides\":[{\"content\":{\"connectorIds\":[\"Out2\",\"In1\"]},\"type\":\"ConnectorPlacement.EquallySpacedRectSide\",\"uuid\":\"a0032173-8ef3-4309-bb40-fe08da9e6df1\"},{\"content\":{\"connectorIds\":[\"In3\",\"Out1\"],\"side\":\"RIGHT\"},\"type\":\"ConnectorPlacement.EquallySpacedRectSide\",\"uuid\":\"9cdcd804-2762-4ca0-b490-38ed7eed87f7\"},{\"content\":{\"connectorIds\":[\"In2\"],\"side\":\"TOP\"},\"type\":\"ConnectorPlacement.EquallySpacedRectSide\",\"uuid\":\"b39ccd24-922c-403c-8220-23b884070dc3\"}]},\"type\":\"ConnectorPlacement.EquallySpacedConnector\",\"uuid\":\"eadb57ab-7193-4630-930c-befd9c6a41f4\"}],\"packageUris\":[\"http://schema.mathworks.com/mf0/Connector/R2020b\"],\"version\":\"1.0\"}"
  Saturation1 : Saturate  UpperLimit=311*0.9*sqrt(1/3)  LowerLimit=-311*0.9*sqrt(1/3)  SampleTime=1e-4
  Scope : Scope  NumInputPorts=2
  Sum1 : Sum  Inputs=|+-
  Sum2 : Sum  Inputs=|+-
  Vd : Outport
  wires:
  A_LESO/2(^i_d) -> Sum1/2, Scope/2
  Gain1/1 -> Sum2/2
  Sum2/1 -> Saturation1/1
  A_LESO/1(^fd_total) -> Gain1/1
  NLESF/1(Out1) -> Sum2/1
  Sum1/1 -> NLESF/1(In1)
  Id_ref/1 -> Sum1/1
  NOB/1(y**) -> A_LESO/2(id_ac)
  id_ac/1 -> NOB/1(y), Scope/1
  NOB/2(OutU) -> Vd/1
  Saturation1/1 -> A_LESO/1(ud), NOB/3(u)

== system ad_pmsm_or/Adapt/Adapt_Iq ==
  Iq_ref : Inport
  iq_ac : Inport  Port=2
  A_LESO : Subsystem
  Gain8 : Gain  Gain=1/bq0
  NLESF : Subsystem
      settings: PortSchema="{\"entries\":[{\"content\":{\"sides\":[{\"content\":{\"connectorIds\":[]},\"type\":\"ConnectorPlacement.EquallySpacedRectSide\",\"uuid\":\"855ad99d-f275-44e1-8b5b-56b977b466e8\"},{\"content\":{\"connectorIds\":[],\"side\":\"RIGHT\"},\"type\":\"ConnectorPlacement.EquallySpacedRectSide\",\"uuid\":\"4b878b09-ea31-423b-8484-bd272f0e87c8\"},{\"content\":{\"connectorIds\":[\"In1\"],\"side\":\"TOP\"},\"type\":\"ConnectorPlacement.EquallySpacedRectSide\",\"uuid\":\"57c50dd4-c343-4c9b-a4ed-e8a0ac5e39c8\"},{\"content\":{\"connectorIds\":[\"Out1\"],\"side\":\"BOTTOM\"},\"type\":\"ConnectorPlacement.EquallySpacedRectSide\",\"uuid\":\"ac7a5b07-13b6-4023-b74a-bbacaa2441c8\"}]},\"type\":\"ConnectorPlacement.EquallySpacedConnector\",\"uuid\":\"c498a5af-adea-4d67-ae4d-0db2496b6d76\"}],\"packageUris\":[\"http://schema.mathworks.com/mf0/Connector/R2020b\"],\"version\":\"1.0\"}"
  NOB : Subsystem
      settings: PortSchema="{\"entries\":[{\"content\":{\"sides\":[{\"content\":{\"connectorIds\":[\"Out2\",\"In1\"]},\"type\":\"ConnectorPlacement.EquallySpacedRectSide\",\"uuid\":\"a0032173-8ef3-4309-bb40-fe08da9e6df1\"},{\"content\":{\"connectorIds\":[\"In3\",\"Out1\"],\"side\":\"RIGHT\"},\"type\":\"ConnectorPlacement.EquallySpacedRectSide\",\"uuid\":\"9cdcd804-2762-4ca0-b490-38ed7eed87f7\"},{\"content\":{\"connectorIds\":[\"In2\"],\"side\":\"TOP\"},\"type\":\"ConnectorPlacement.EquallySpacedRectSide\",\"uuid\":\"b39ccd24-922c-403c-8220-23b884070dc3\"}]},\"type\":\"ConnectorPlacement.EquallySpacedConnector\",\"uuid\":\"eadb57ab-7193-4630-930c-befd9c6a41f4\"}],\"packageUris\":[\"http://schema.mathworks.com/mf0/Connector/R2020b\"],\"version\":\"1.0\"}"
  Saturation2 : Saturate  UpperLimit=311*0.9*sqrt(1/3)  LowerLimit=-311*0.9*sqrt(1/3)  SampleTime=1e-4
  Scope : Scope  NumInputPorts=2
  Sum3 : Sum  Inputs=|+-
  Sum4 : Sum  Inputs=|+-
  Vq : Outport
  wires:
  NLESF/1(Out1) -> Sum4/1
  Sum3/1 -> NLESF/1(In1)
  A_LESO/1(^fq_total) -> Gain8/1
  Iq_ref/1 -> Sum3/1
  Sum4/1 -> Saturation2/1
  Gain8/1 -> Sum4/2
  A_LESO/2(^i_q) -> Sum3/2, Scope/2
  iq_ac/1 -> Scope/1, NOB/1(y)
  NOB/1(y**) -> A_LESO/2(iq_ac)
  NOB/2(OutU) -> Vq/1
  Saturation2/1 -> NOB/3(u), A_LESO/1(uq)

== system ad_pmsm_or/Adapt/Anti_Park ==
  Vq : Inport
  Vd : Inport  Port=2
  Fcn : Fcn  Expr=cos(u[1])*u[2]-sin(u[1])*u[3]
  Fcn1 : Fcn  Expr=sin(u[1])*u[2]+cos(u[1])*u[3]
  Mux1 : Mux  Inputs=3
  Ualpha : Outport
  Ubeta : Outport  Port=2
  wires:
  Fcn1/1 -> Ubeta/1
  Fcn/1 -> Ualpha/1
  Mux1/1 -> Fcn/1, Fcn1/1
  Vd/1 -> Mux1/2
  Vq/1 -> Mux1/3
  [The3] -> Mux1/1

== system ad_pmsm_or/Adapt/Clark ==
  A : Inport
  B : Inport  Port=2
  C : Inport  Port=3
  Mux : Mux  Inputs=3
  alpha : Fcn  Expr=(u(1)-0.5*(u(2)+u(3)))*2/3
  beta : Fcn  Expr=sqrt(3)/2*(u(2)-u(3))*2/3
  Alpha : Outport
  Beta : Outport  Port=2
  wires:
  alpha/1 -> Alpha/1
  B/1 -> Mux/2
  C/1 -> Mux/3
  A/1 -> Mux/1
  Mux/1 -> beta/1, alpha/1
  beta/1 -> Beta/1

== system ad_pmsm_or/Adapt/Mux ==
  m : Inport
  Bus Selector : BusSelector  OutputSignals=Stator current is_a (A),Stator current is_b (A),Stator current is_c (A)
  Bus Selector1 : BusSelector  OutputSignals=Rotor speed wm (rad/s),Rotor angle thetam (rad),Electromagnetic torque Te (N*m)
  Mux : Mux  Inputs=3
  Te : Outport
  The : Outport  Port=2
  Iabc2 : Outport  Port=3
  Wm : Outport  Port=4
  wires:
  Bus Selector1/1 -> Wm/1  "<Rotor speed wm (rad/s)>"
  Bus Selector1/2 -> The/1  "<Rotor angle thetam (rad)>"
  Bus Selector1/3 -> Te/1  "<Electromagnetic torque Te (N*m)>"
  m/1 -> Bus Selector/1, Bus Selector1/1
  Bus Selector/2 -> Mux/2  "<Stator current is_b (A)>"
  Bus Selector/3 -> Mux/3  "<Stator current is_c (A)>"
  Bus Selector/1 -> Mux/1  "<Stator current is_a (A)>"
  Mux/1 -> Iabc2/1

== system ad_pmsm_or/Adapt/Plark ==
  Alpha : Inport
  Beta : Inport  Port=2
  The3 : Inport  Port=3
  Add : Sum
  Add1 : Sum
  Band-Limited White Noise1 : simulink/Sources/Band-Limited White Noise  Cov=[0.0001]  Ts=0.0001  seed=[23341]
  Mux : Mux  Inputs=3
  Sine Wave3 : Sin  Amplitude=0.5  Frequency=350*2*pi  SampleTime=0
  d : Fcn  Expr=u(1)*cos(u(3))+u(2)*sin(u(3))
  q : Fcn  Expr=-u(1)*sin(u(3))+u(2)*cos(u(3))
  D : Outport
  Q : Outport  Port=2
  wires:
  Beta/1 -> Mux/2
  Alpha/1 -> Mux/1
  Mux/1 -> q/1, d/1
  The3/1 -> Mux/3
  d/1 -> Add/2
  Add/1 -> D/1
  Add1/1 -> Q/1
  q/1 -> Add1/2

== system ad_pmsm_or/Adapt/SVPWM ==
  Valpha : Inport
  Vbeta : Inport  Port=2
  PWM : Subsystem
  Repeating Sequence : simulink/Sources/Repeating Sequence  rep_seq_t=[0 0.00005 0.0001]  rep_seq_y=[0 0.00005 0]
  Sector Caculate : Subsystem
  T1T1 Caculate : Subsystem
  Tcm Caculate : Subsystem
  Tpwm : Constant  Value=0.0001
  Vdc : Constant  Value=311
  XYZ Caculate : Subsystem
  pulse : Outport
  wires:
  PWM/1(PWM) -> pulse/1
  Repeating Sequence/1 -> PWM/1(In)
  Vbeta/1 -> XYZ Caculate/2(Ubeta), Sector Caculate/2(Ubeta)
  T1T1 Caculate/1(T1) -> Tcm Caculate/2(T1)
  Valpha/1 -> XYZ Caculate/1(Ualpha), Sector Caculate/1(Ualpha)
  T1T1 Caculate/2(T2) -> Tcm Caculate/3(T2)
  Sector Caculate/1("N ") -> Tcm Caculate/1(N), T1T1 Caculate/1(N)
  XYZ Caculate/1(XYZ) -> T1T1 Caculate/2(XYZ)
  Tpwm/1 -> XYZ Caculate/3(Ts), Tcm Caculate/4(Tpwm), T1T1 Caculate/3(Tpwm)
  Vdc/1 -> XYZ Caculate/4(Udc)
  Tcm Caculate/1(Tcm1 Tcm2 Tcm3) -> PWM/2(Tcm123)

== system ad_pmsm_or/Adapt/Speed ==
  note: Discrete PID Controller
  note: Pierre Giroux, Gilbert Sybille
      | Power System Simulation Laboratory
      | IREQ, Hydro-Quebc
  Error : Inport  SampleTime=Ts
  Discrete-Time Integrator : DiscreteIntegrator  InitialCondition=Init  SampleTime=Ts  LimitOutput=on  UpperSaturationLimit=UpperLimit  LowerSaturationLimit=LowerLimit  ICPrevOutput=DiscIntNeverNeededParam  ICPrevScaledInput=DiscIntNeverNeededParam
  Kp1 : Gain  Gain=Ba  SaturateOnIntegerOverflow=on  SampleTime=Ts  OutDataTypeStr=Inherit: Same as input  ParamDataTypeStr=Inherit: Same as input
  Kp4 : Gain  Gain=Kpw  SaturateOnIntegerOverflow=on  SampleTime=Ts  OutDataTypeStr=Inherit: Same as input  ParamDataTypeStr=Inherit: Same as input
  Kp5 : Gain  Gain=Kiw  SaturateOnIntegerOverflow=on  SampleTime=Ts  OutDataTypeStr=Inherit: Same as input  ParamDataTypeStr=Inherit: Same as input
  Saturation2 : Saturate  UpperLimit=UpperLimit  LowerLimit=LowerLimit  SampleTime=Ts
  Sum6 : Sum  Inputs=++-  InputSameDT=on  SaturateOnIntegerOverflow=on  SampleTime=Ts  OutDataTypeStr=Inherit: Same as first input
  Zero-Order Hold : ZeroOrderHold  SampleTime=Ts
  Out : Outport  SampleTime=Ts  InitialOutput=0
  wires:
  Error/1 -> Kp1/1, Kp5/1, Kp4/1
  Zero-Order Hold/1 -> Sum6/1
  Saturation2/1 -> Out/1
  Discrete-Time Integrator/1 -> Sum6/2
  Kp4/1 -> Zero-Order Hold/1
  Kp5/1 -> Discrete-Time Integrator/1
  Sum6/1 -> Saturation2/1
  Kp1/1 -> Sum6/3

== system ad_pmsm_or/LADRC/Anti_Park ==
  Vq : Inport
  Vd : Inport  Port=2
  Fcn : Fcn  Expr=cos(u[1])*u[2]-sin(u[1])*u[3]
  Fcn1 : Fcn  Expr=sin(u[1])*u[2]+cos(u[1])*u[3]
  Mux1 : Mux  Inputs=3
  Ualpha : Outport
  Ubeta : Outport  Port=2
  wires:
  Fcn1/1 -> Ubeta/1
  Fcn/1 -> Ualpha/1
  Mux1/1 -> Fcn/1, Fcn1/1
  Vd/1 -> Mux1/2
  Vq/1 -> Mux1/3
  [The2] -> Mux1/1

== system ad_pmsm_or/LADRC/Clark ==
  A : Inport
  B : Inport  Port=2
  C : Inport  Port=3
  Mux : Mux  Inputs=3
  alpha : Fcn  Expr=(u(1)-0.5*(u(2)+u(3)))*2/3
  beta : Fcn  Expr=sqrt(3)/2*(u(2)-u(3))*2/3
  Alpha : Outport
  Beta : Outport  Port=2
  wires:
  alpha/1 -> Alpha/1
  B/1 -> Mux/2
  C/1 -> Mux/3
  A/1 -> Mux/1
  Mux/1 -> beta/1, alpha/1
  beta/1 -> Beta/1

== system ad_pmsm_or/LADRC/LADRC_Id ==
  Id_ref : Inport
  id_ac : Inport  Port=2
  Discrete Transfer Fcn : DiscreteTransferFcn  Numerator=[0.237 0.237]  Denominator=[1 -0.522]  SampleTime=1e-4
  Gain8 : Gain  Gain=1/b0_d
  LESO : Subsystem
  NLESF : Subsystem
      settings: PortSchema="{\"entries\":[{\"content\":{\"sides\":[{\"content\":{\"connectorIds\":[]},\"type\":\"ConnectorPlacement.EquallySpacedRectSide\",\"uuid\":\"855ad99d-f275-44e1-8b5b-56b977b466e8\"},{\"content\":{\"connectorIds\":[],\"side\":\"RIGHT\"},\"type\":\"ConnectorPlacement.EquallySpacedRectSide\",\"uuid\":\"4b878b09-ea31-423b-8484-bd272f0e87c8\"},{\"content\":{\"connectorIds\":[\"In1\"],\"side\":\"TOP\"},\"type\":\"ConnectorPlacement.EquallySpacedRectSide\",\"uuid\":\"57c50dd4-c343-4c9b-a4ed-e8a0ac5e39c8\"},{\"content\":{\"connectorIds\":[\"Out1\"],\"side\":\"BOTTOM\"},\"type\":\"ConnectorPlacement.EquallySpacedRectSide\",\"uuid\":\"ac7a5b07-13b6-4023-b74a-bbacaa2441c8\"}]},\"type\":\"ConnectorPlacement.EquallySpacedConnector\",\"uuid\":\"c498a5af-adea-4d67-ae4d-0db2496b6d76\"}],\"packageUris\":[\"http://schema.mathworks.com/mf0/Connector/R2020b\"],\"version\":\"1.0\"}"
  Saturation2 : Saturate  UpperLimit=311*0.9*sqrt(1/3)  LowerLimit=-311*0.9*sqrt(1/3)  SampleTime=1e-4
  Scope : Scope
  Sum3 : Sum  Inputs=|+-
  Sum4 : Sum  Inputs=|+-
  Vd : Outport
  wires:
  Saturation2/1 -> Vd/1
  NLESF/1(Out1) -> Sum4/1
  Sum3/1 -> NLESF/1(In1)
  LESO/1(f) -> Gain8/1
  Id_ref/1 -> Sum3/1
  Sum4/1 -> LESO/1(u), Saturation2/1
  LESO/2(z) -> Sum3/2
  id_ac/1 -> LESO/2(y)
  Gain8/1 -> Scope/1, Sum4/2

== system ad_pmsm_or/LADRC/LADRC_Iq ==
  Iq_ref : Inport
  iq_ac : Inport  Port=2
  Discrete Transfer Fcn : DiscreteTransferFcn  Numerator=[0.237 0.237]  Denominator=[1 -0.522]  SampleTime=1e-4
  Gain8 : Gain  Gain=1/b0_q
  LESO : Subsystem
  NLESF : Subsystem
      settings: PortSchema="{\"entries\":[{\"content\":{\"sides\":[{\"content\":{\"connectorIds\":[]},\"type\":\"ConnectorPlacement.EquallySpacedRectSide\",\"uuid\":\"855ad99d-f275-44e1-8b5b-56b977b466e8\"},{\"content\":{\"connectorIds\":[],\"side\":\"RIGHT\"},\"type\":\"ConnectorPlacement.EquallySpacedRectSide\",\"uuid\":\"4b878b09-ea31-423b-8484-bd272f0e87c8\"},{\"content\":{\"connectorIds\":[\"In1\"],\"side\":\"TOP\"},\"type\":\"ConnectorPlacement.EquallySpacedRectSide\",\"uuid\":\"57c50dd4-c343-4c9b-a4ed-e8a0ac5e39c8\"},{\"content\":{\"connectorIds\":[\"Out1\"],\"side\":\"BOTTOM\"},\"type\":\"ConnectorPlacement.EquallySpacedRectSide\",\"uuid\":\"ac7a5b07-13b6-4023-b74a-bbacaa2441c8\"}]},\"type\":\"ConnectorPlacement.EquallySpacedConnector\",\"uuid\":\"c498a5af-adea-4d67-ae4d-0db2496b6d76\"}],\"packageUris\":[\"http://schema.mathworks.com/mf0/Connector/R2020b\"],\"version\":\"1.0\"}"
  Saturation2 : Saturate  UpperLimit=311*0.9*sqrt(1/3)  LowerLimit=-311*0.9*sqrt(1/3)  SampleTime=1e-4
  Scope : Scope  NumInputPorts=2
  Scope1 : Scope
  Sum3 : Sum  Inputs=|+-
  Sum4 : Sum  Inputs=|+-
  Vq : Outport
  wires:
  Saturation2/1 -> Vq/1
  NLESF/1(Out1) -> Sum4/1
  Sum3/1 -> NLESF/1(In1)
  LESO/1(f) -> Gain8/1
  Iq_ref/1 -> Sum3/1
  Sum4/1 -> LESO/1(u), Saturation2/1
  LESO/2(z) -> Scope/2, Sum3/2
  iq_ac/1 -> Scope/1, LESO/2(y)
  Gain8/1 -> Scope1/1, Sum4/2

== system ad_pmsm_or/LADRC/LADRC_SPEED ==
  V_ref : Inport
  V_ac : Inport  Port=2
  Gain8 : Gain  Gain=1/b0_V
  LESO : Subsystem
  NLESF : Subsystem
      settings: PortSchema="{\"entries\":[{\"content\":{\"sides\":[{\"content\":{\"connectorIds\":[]},\"type\":\"ConnectorPlacement.EquallySpacedRectSide\",\"uuid\":\"855ad99d-f275-44e1-8b5b-56b977b466e8\"},{\"content\":{\"connectorIds\":[],\"side\":\"RIGHT\"},\"type\":\"ConnectorPlacement.EquallySpacedRectSide\",\"uuid\":\"4b878b09-ea31-423b-8484-bd272f0e87c8\"},{\"content\":{\"connectorIds\":[\"In1\"],\"side\":\"TOP\"},\"type\":\"ConnectorPlacement.EquallySpacedRectSide\",\"uuid\":\"57c50dd4-c343-4c9b-a4ed-e8a0ac5e39c8\"},{\"content\":{\"connectorIds\":[\"Out1\"],\"side\":\"BOTTOM\"},\"type\":\"ConnectorPlacement.EquallySpacedRectSide\",\"uuid\":\"ac7a5b07-13b6-4023-b74a-bbacaa2441c8\"}]},\"type\":\"ConnectorPlacement.EquallySpacedConnector\",\"uuid\":\"c498a5af-adea-4d67-ae4d-0db2496b6d76\"}],\"packageUris\":[\"http://schema.mathworks.com/mf0/Connector/R2020b\"],\"version\":\"1.0\"}"
  Saturation2 : Saturate  UpperLimit=8  LowerLimit=-8  SampleTime=1e-4
  Sum3 : Sum  Inputs=|+-
  Sum4 : Sum  Inputs=|+-
  iq : Outport
  wires:
  Saturation2/1 -> iq/1
  NLESF/1(Out1) -> Sum4/1
  Sum3/1 -> NLESF/1(In1)
  LESO/1(f) -> Gain8/1
  V_ref/1 -> Sum3/1
  Sum4/1 -> LESO/1(u), Saturation2/1
  Gain8/1 -> Sum4/2
  LESO/2(z) -> Sum3/2
  V_ac/1 -> LESO/2(y)

== system ad_pmsm_or/LADRC/Mux ==
  m : Inport
  Bus Selector : BusSelector  OutputSignals=Stator current is_a (A),Stator current is_b (A),Stator current is_c (A)
  Bus Selector1 : BusSelector  OutputSignals=Rotor speed wm (rad/s),Rotor angle thetam (rad),Electromagnetic torque Te (N*m)
  Mux : Mux  Inputs=3
  Te : Outport
  The : Outport  Port=2
  Iabc2 : Outport  Port=3
  Wm : Outport  Port=4
  wires:
  Bus Selector1/1 -> Wm/1  "<Rotor speed wm (rad/s)>"
  Bus Selector1/2 -> The/1  "<Rotor angle thetam (rad)>"
  Bus Selector1/3 -> Te/1  "<Electromagnetic torque Te (N*m)>"
  m/1 -> Bus Selector/1, Bus Selector1/1
  Bus Selector/2 -> Mux/2  "<Stator current is_b (A)>"
  Bus Selector/3 -> Mux/3  "<Stator current is_c (A)>"
  Bus Selector/1 -> Mux/1  "<Stator current is_a (A)>"
  Mux/1 -> Iabc2/1

== system ad_pmsm_or/LADRC/Plark ==
  Alpha : Inport
  Beta : Inport  Port=2
  The2 : Inport  Port=3
  Add : Sum
  Add1 : Sum
  Band-Limited White Noise1 : simulink/Sources/Band-Limited White Noise  Cov=[0.0001]  Ts=0.0001  seed=[23341]
  Mux : Mux  Inputs=3
  Sine Wave3 : Sin  Amplitude=0.5  Frequency=200*2*pi  SampleTime=0
  d : Fcn  Expr=u(1)*cos(u(3))+u(2)*sin(u(3))
  q : Fcn  Expr=-u(1)*sin(u(3))+u(2)*cos(u(3))
  D : Outport
  Q : Outport  Port=2
  wires:
  Beta/1 -> Mux/2
  Alpha/1 -> Mux/1
  Mux/1 -> q/1, d/1
  The2/1 -> Mux/3
  Add/1 -> D/1
  d/1 -> Add/2
  Add1/1 -> Q/1
  q/1 -> Add1/2
  Band-Limited White Noise1/1 -> Add1/1, Add/1

== system ad_pmsm_or/LADRC/SVPWM ==
  Valpha : Inport
  Vbeta : Inport  Port=2
  PWM : Subsystem
  Repeating Sequence : simulink/Sources/Repeating Sequence  rep_seq_t=[0 0.00005 0.0001]  rep_seq_y=[0 0.00005 0]
  Sector Caculate : Subsystem
  T1T1 Caculate : Subsystem
  Tcm Caculate : Subsystem
  Tpwm : Constant  Value=0.0001
  Vdc : Constant  Value=311
  XYZ Caculate : Subsystem
  pulse : Outport
  wires:
  PWM/1(PWM) -> pulse/1
  Repeating Sequence/1 -> PWM/1(In)
  Vbeta/1 -> XYZ Caculate/2(Ubeta), Sector Caculate/2(Ubeta)
  T1T1 Caculate/1(T1) -> Tcm Caculate/2(T1)
  Valpha/1 -> XYZ Caculate/1(Ualpha), Sector Caculate/1(Ualpha)
  T1T1 Caculate/2(T2) -> Tcm Caculate/3(T2)
  Sector Caculate/1("N ") -> Tcm Caculate/1(N), T1T1 Caculate/1(N)
  XYZ Caculate/1(XYZ) -> T1T1 Caculate/2(XYZ)
  Tpwm/1 -> XYZ Caculate/3(Ts), Tcm Caculate/4(Tpwm), T1T1 Caculate/3(Tpwm)
  Vdc/1 -> XYZ Caculate/4(Udc)
  Tcm Caculate/1(Tcm1 Tcm2 Tcm3) -> PWM/2(Tcm123)

== system ad_pmsm_or/LADRC/Speed ==
  note: Discrete PID Controller
  note: Pierre Giroux, Gilbert Sybille
      | Power System Simulation Laboratory
      | IREQ, Hydro-Quebc
  Error : Inport  SampleTime=Ts
  Discrete-Time Integrator : DiscreteIntegrator  InitialCondition=Init  SampleTime=Ts  LimitOutput=on  UpperSaturationLimit=UpperLimit  LowerSaturationLimit=LowerLimit  ICPrevOutput=DiscIntNeverNeededParam  ICPrevScaledInput=DiscIntNeverNeededParam
  Kp1 : Gain  Gain=Ba  SaturateOnIntegerOverflow=on  SampleTime=Ts  OutDataTypeStr=Inherit: Same as input  ParamDataTypeStr=Inherit: Same as input
  Kp4 : Gain  Gain=Kpw  SaturateOnIntegerOverflow=on  SampleTime=Ts  OutDataTypeStr=Inherit: Same as input  ParamDataTypeStr=Inherit: Same as input
  Kp5 : Gain  Gain=Kiw  SaturateOnIntegerOverflow=on  SampleTime=Ts  OutDataTypeStr=Inherit: Same as input  ParamDataTypeStr=Inherit: Same as input
  Saturation2 : Saturate  UpperLimit=UpperLimit  LowerLimit=LowerLimit  SampleTime=Ts
  Sum6 : Sum  Inputs=++-  InputSameDT=on  SaturateOnIntegerOverflow=on  SampleTime=Ts  OutDataTypeStr=Inherit: Same as first input
  Zero-Order Hold : ZeroOrderHold  SampleTime=Ts
  Out : Outport  SampleTime=Ts  InitialOutput=0
  wires:
  Error/1 -> Kp1/1, Kp5/1, Kp4/1
  Zero-Order Hold/1 -> Sum6/1
  Saturation2/1 -> Out/1
  Discrete-Time Integrator/1 -> Sum6/2
  Kp4/1 -> Zero-Order Hold/1
  Kp5/1 -> Discrete-Time Integrator/1
  Sum6/1 -> Saturation2/1
  Kp1/1 -> Sum6/3

== system ad_pmsm_or/LADRC/定时开关 ==
  In1 : Inport
  Product2 : Product
  Step : Step  Time=0.3  SampleTime=0
  Out1 : Outport
  wires:
  Step/1 -> Product2/2
  In1/1 -> Product2/1
  Product2/1 -> Out1/1

== system ad_pmsm_or/NOB_LADRC/Anti_Park ==
  Vq : Inport
  Vd : Inport  Port=2
  Fcn : Fcn  Expr=cos(u[1])*u[2]-sin(u[1])*u[3]
  Fcn1 : Fcn  Expr=sin(u[1])*u[2]+cos(u[1])*u[3]
  Mux1 : Mux  Inputs=3
  Ualpha : Outport
  Ubeta : Outport  Port=2
  wires:
  Fcn1/1 -> Ubeta/1
  Fcn/1 -> Ualpha/1
  Mux1/1 -> Fcn/1, Fcn1/1
  Vd/1 -> Mux1/2
  Vq/1 -> Mux1/3
  [The4] -> Mux1/1

== system ad_pmsm_or/NOB_LADRC/Clark ==
  A : Inport
  B : Inport  Port=2
  C : Inport  Port=3
  Mux : Mux  Inputs=3
  alpha : Fcn  Expr=(u(1)-0.5*(u(2)+u(3)))*2/3
  beta : Fcn  Expr=sqrt(3)/2*(u(2)-u(3))*2/3
  Alpha : Outport
  Beta : Outport  Port=2
  wires:
  alpha/1 -> Alpha/1
  B/1 -> Mux/2
  C/1 -> Mux/3
  A/1 -> Mux/1
  Mux/1 -> beta/1, alpha/1
  beta/1 -> Beta/1

== system ad_pmsm_or/NOB_LADRC/LADRC_Id ==
  Id_ref : Inport
  id_ac : Inport  Port=2
  Gain8 : Gain  Gain=1/b0_d
  LESO : Subsystem
  NLESF : Subsystem
      settings: PortSchema="{\"entries\":[{\"content\":{\"sides\":[{\"content\":{\"connectorIds\":[]},\"type\":\"ConnectorPlacement.EquallySpacedRectSide\",\"uuid\":\"855ad99d-f275-44e1-8b5b-56b977b466e8\"},{\"content\":{\"connectorIds\":[],\"side\":\"RIGHT\"},\"type\":\"ConnectorPlacement.EquallySpacedRectSide\",\"uuid\":\"4b878b09-ea31-423b-8484-bd272f0e87c8\"},{\"content\":{\"connectorIds\":[\"In1\"],\"side\":\"TOP\"},\"type\":\"ConnectorPlacement.EquallySpacedRectSide\",\"uuid\":\"57c50dd4-c343-4c9b-a4ed-e8a0ac5e39c8\"},{\"content\":{\"connectorIds\":[\"Out1\"],\"side\":\"BOTTOM\"},\"type\":\"ConnectorPlacement.EquallySpacedRectSide\",\"uuid\":\"ac7a5b07-13b6-4023-b74a-bbacaa2441c8\"}]},\"type\":\"ConnectorPlacement.EquallySpacedConnector\",\"uuid\":\"c498a5af-adea-4d67-ae4d-0db2496b6d76\"}],\"packageUris\":[\"http://schema.mathworks.com/mf0/Connector/R2020b\"],\"version\":\"1.0\"}"
  NOB1 : Subsystem
      settings: PortSchema="{\"entries\":[{\"content\":{\"sides\":[{\"content\":{\"connectorIds\":[\"Out2\",\"In1\"]},\"type\":\"ConnectorPlacement.EquallySpacedRectSide\",\"uuid\":\"a0032173-8ef3-4309-bb40-fe08da9e6df1\"},{\"content\":{\"connectorIds\":[\"In3\",\"Out1\"],\"side\":\"RIGHT\"},\"type\":\"ConnectorPlacement.EquallySpacedRectSide\",\"uuid\":\"9cdcd804-2762-4ca0-b490-38ed7eed87f7\"},{\"content\":{\"connectorIds\":[\"In2\"],\"side\":\"TOP\"},\"type\":\"ConnectorPlacement.EquallySpacedRectSide\",\"uuid\":\"b39ccd24-922c-403c-8220-23b884070dc3\"}]},\"type\":\"ConnectorPlacement.EquallySpacedConnector\",\"uuid\":\"eadb57ab-7193-4630-930c-befd9c6a41f4\"}],\"packageUris\":[\"http://schema.mathworks.com/mf0/Connector/R2020b\"],\"version\":\"1.0\"}"
  Saturation2 : Saturate  UpperLimit=311*0.9*sqrt(1/3)  LowerLimit=-311*0.9*sqrt(1/3)  SampleTime=1e-4
  Scope : Scope
  Sum3 : Sum  Inputs=|+-
  Sum4 : Sum  Inputs=-++-
  Vd : Outport
  wires:
  Sum3/1 -> NLESF/1(In1)
  LESO/1(f) -> Gain8/1
  Id_ref/1 -> Sum3/1
  LESO/2(z) -> Sum3/2
  Sum4/1 -> Saturation2/1, LESO/1(u)
  Gain8/1 -> Scope/1, Sum4/4
  NLESF/1(Out1) -> Sum4/3
  NOB1/2(OutU) -> Vd/1
  Saturation2/1 -> NOB1/3(u)
  NOB1/1(y**) -> LESO/2(y)
  id_ac/1 -> NOB1/1(y)
